simulink model "QPSK_vold"  (R2015a)
settings: Solver=ode3  SolverMode=SingleTasking  StartTime=0.0  StopTime=1  FixedStep=1e-3  RelTol=1e-3
libraries: simulink x2, commdigbbndpm3 x1, commrandsrc2 x1
settings Model: CovMetricSettings=dwe  CovHtmlReporting=off  covSaveCumulativeToWorkspaceVar=off  CovSaveSingleToWorkspaceVar=off  CovExternalEMLEnable=on  Creator=marcone  LastModifiedBy=marcone
settings DataIOCC: LimitDataPoints=off  SaveFormat=Dataset
settings DebuggingCC: SFUnexpectedBacktrackingDiag=error  SFNoUnconditionalDefaultTransitionDiag=error
settings HardwareCC: ProdBitPerPointer=64  ProdLargestAtomicFloat=Float  ProdIntDivRoundTo=Zero  ProdEndianess=LittleEndian  ProdHWDeviceType=Specified
settings ModelReferenceCC: PropagateSignalLabelsOutOfModel=on
settings SFSimCC: SimUseLocalCustomCode=on
settings RTWCC: RTWUseLocalCustomCode=on
settings GRTTargetCC: TargetLangStandard=C99 (ISO)  GeneratePreprocessorConditionals=Use local settings

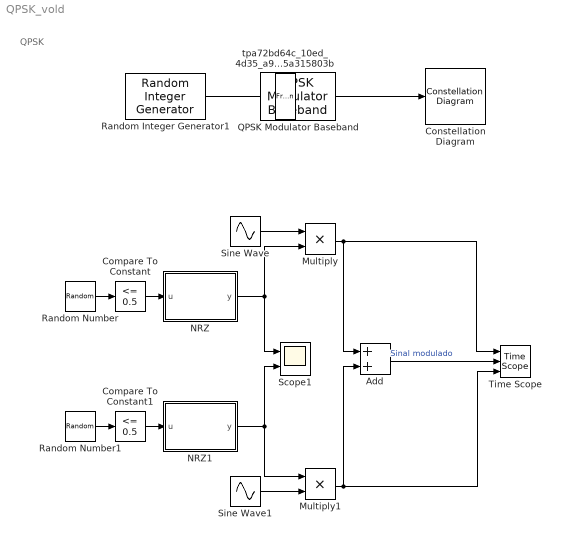
== system QPSK_vold ==
  note: QPSK
  Add : Sum
  Compare To Constant : simulink/Logic and Bit Operations/Compare To Constant  relop=<=  const=0.5  OutDataTypeStr=boolean
  Compare To Constant1 : simulink/Logic and Bit Operations/Compare To Constant  relop=<=  const=0.5  OutDataTypeStr=boolean
  Constellation Diagram : ConstellationDiagram
  Multiply : Product
  Multiply1 : Product
  NRZ : MATLAB Function  TreatAsAtomicUnit=on
      settings: PermitHierarchicalResolution=ParametersOnly
  NRZ1 : MATLAB Function  TreatAsAtomicUnit=on
      settings: PermitHierarchicalResolution=ParametersOnly
  QPSK Modulator Baseband : commdigbbndpm3/QPSK Modulator Baseband  InType=Integer  Enc=Gray  Ph=pi/4  outDtype=double  outWordLen=16  outUDDataType=sfix(16)  outFracLenMode=Best precision  outFracLen=15
  Random Number : RandomNumber  Mean=0.5  SampleTime=0.1
  Random Number1 : RandomNumber  Mean=0.5  Seed=10  SampleTime=0.1
  Random Integer Generator1 : commrandsrc2/Random Integer Generator  mul=4  seed=0  Ts=1  sampPerFrame=10000  outDataType=double  frameBased=on
  Scope1 : Scope  NumInputPorts=2
      settings: TimeRange=auto  MaxDataPoints=5000  SaveToWorkspace=off  SaveName=ScopeData  YMin=-1.25~-1.25  YMax=1.25~1.25  SampleTime=-1
  Sine Wave : Sin  Amplitude=2  Frequency=500  SampleTime=0
  Sine Wave1 : Sin  Amplitude=2  Frequency=500  Phase=90*pi/180  SampleTime=0
  Time Scope : TimeScope  DefaultConfigurationName=spbscopes.TimeScopeBlockCfg  NumInputPorts=3
  tpa72bd64c_10ed_4d35_a9ab_2595a315803b : FrameConversion  OutFrame=Sample-based
  wires:
  Compare To Constant/1 -> NRZ/1(u)
  Compare To Constant1/1 -> NRZ1/1(u)
  NRZ/1(y) -> Multiply/2, Scope1/1
  NRZ1/1(y) -> Multiply1/1, Scope1/2
  Random Number/1 -> Compare To Constant/1
  Random Number1/1 -> Compare To Constant1/1
  Sine Wave/1 -> Multiply/1
  Multiply/1 -> Time Scope/1, Add/1
  Multiply1/1 -> Time Scope/3, Add/2
  Sine Wave1/1 -> Multiply1/2
  Add/1 -> Time Scope/2  "Sinal modulado"
  QPSK Modulator Baseband/1 -> Constellation Diagram/1
  Random Integer Generator1/1 -> tpa72bd64c_10ed_4d35_a9ab_2595a315803b/1
  tpa72bd64c_10ed_4d35_a9ab_2595a315803b/1 -> QPSK Modulator Baseband/1

== matlab function QPSK_vold/NRZ1 ==
  data: u input; y output
function y = fcn(u)
if u == 1
    y = 1;
else
    y = -1;
end
end

== matlab function QPSK_vold/NRZ ==
  data: u input; y output
function y = fcn(u)
if u == 1
    y = 1;
else
    y = -1;
end
end
